simulink model "Commande_voiture_versionFinale2019"  (R2019b)
settings: Solver=ode1  StartTime=0.0  StopTime=inf  FixedStep=0.002  RelTol=1e-3  EnableMultiTasking=on
libraries: simulink x2, arduinolib x1
settings Model: SimulationMode=external  ExtModeTrigDuration=2  Creator=Alex  LastModifiedBy=franc
settings SolverCC: AutoInsertRateTranBlk=on
settings DataIOCC: SaveFormat=StructureWithTime  ReturnWorkspaceOutputs=off
settings OptimizationCC: PassReuseOutputArgsAs=Individual arguments  MaxStackSize=64  EfficientTunableParamExpr=on
settings DebuggingCC: ParameterPrecisionLossMsg=none  ParameterTunabilityLossMsg=error  ArithmeticOperatorsInVariantConditions=warning
settings HardwareCC: ProdBitPerInt=16  ProdBitPerPointer=16  ProdBitPerSizeT=16  ProdBitPerPtrDiffT=16  ProdLargestAtomicFloat=None  ProdWordSize=8  ProdHWDeviceType=Atmel->AVR
settings SFSimCC: SimUseLocalCustomCode=off  MATLABDynamicMemAlloc=off  CustomCodeUndefinedFunction=UseInterfaceOnly
settings RTWCC: SystemTargetFile=ert.tlc  HardwareBoard=Arduino Mega 2560  TLCOptions=-aInlineSetEventsForThisBaseRateFcn=TLC_FALSE -aSuppressMultiTaskScheduler=TLC_FALSE -aRateBasedStepFcn=1  TemplateMakefile=ert_default_tmf  RTWUseLocalCustomCode=off  Toolchain=Arduino AVR  BuildConfiguration=Faster Runs  IncludeHyperlinkInReport=on
settings CodeAppCC: ForceParamTrailComments=on  IgnoreCustomStorageClasses=off  OperatorAnnotations=on  SimulinkDataObjDesc=on  SFDataObjDesc=on  InsertBlockDesc=on
settings ERTTargetCC: SupportContinuousTime=on  SupportVariableSizeSignals=on

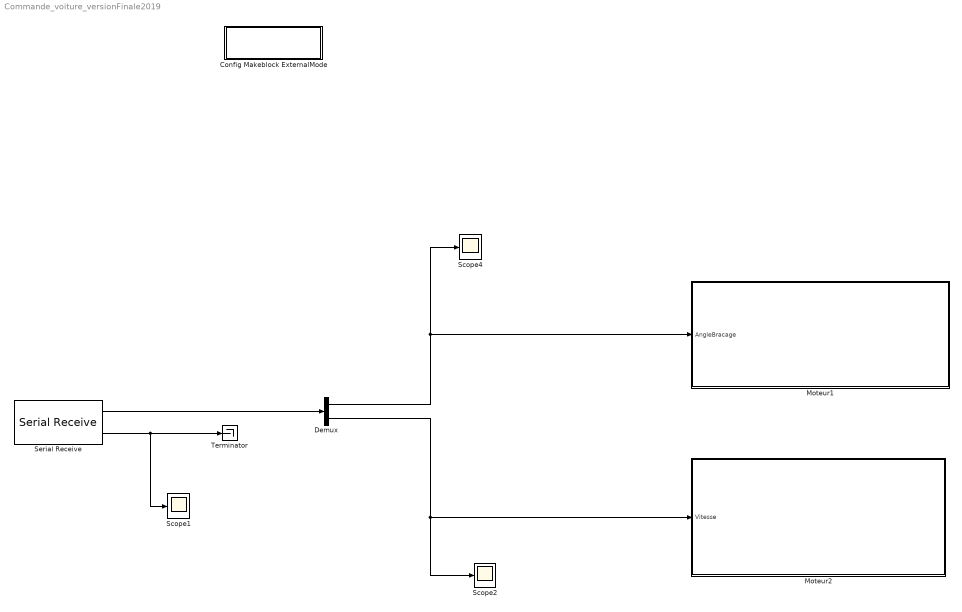
== system Commande_voiture_versionFinale2019 ==
  Config Makeblock ExternalMode : Subsystem  LoadFcn=set_param(gcb,'MaskHideContents','on')  InitFcn=|  TreatAsAtomicUnit=on
      | codertarget.arduinobase.registry.setBaudRate(gcs,115200)
      | set_param(gcb,'MaskHideContents','on')
      mask Display: disp('Makeblock external mode')
  Demux : Demux  Outputs=2
  Moteur1 : Subsystem
  Moteur2 : Subsystem
  Scope1 : Scope
  Scope2 : Scope
  Scope4 : Scope
  Serial Receive : arduinolib/Serial Receive  isARMArch=off  portNumber=2  DataType=int8  Datalength=2  SampleTime=0.1  showOutStatus=on  blockPlatform=arduino
      settings: SourceProductBaseCode=ARDUINO
  Terminator : Terminator
  wires:
  Serial Receive/2 -> Terminator/1, Scope1/1
  Serial Receive/1 -> Demux/1
  Demux/2 -> Scope2/1, Moteur2/1(Vitesse)
  Demux/1 -> Scope4/1, Moteur1/1(AngleBracage)

== system Commande_voiture_versionFinale2019/Config Makeblock ExternalMode ==

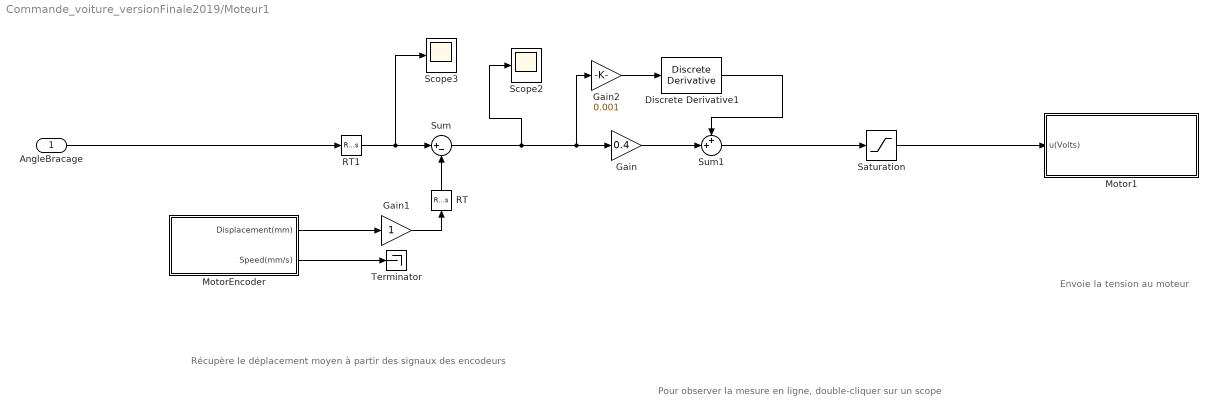
== system Commande_voiture_versionFinale2019/Moteur1 ==
  note: Pour observer la mesure en ligne, double-cliquer sur un scope
  note: Envoie la tension au moteur
  note: Récupère le déplacement moyen à partir des signaux des encodeurs
  AngleBracage : Inport
  Discrete Derivative1 : simulink/Discrete/Discrete Derivative  gainval=1.0  ICPrevScaledInput=0.0  OutMin=[]  OutMax=[]  OutDataType=fixdt(1, 16)  OutScaling=2^-10  DoSatur=off
  Gain : Gain  Gain=0.4
  Gain1 : Gain
  Gain2 : Gain  Gain=0.001
  Motor1 : Subsystem  mask{Vmax=12}
      mask prompts: Vmax "Power supply Voltage"
  MotorEncoder : Subsystem  mask{pulsePerTurn=8, beltPitch=1, nTeeth=40, gearRatio=75}
      mask prompts: pulsePerTurn "Encoder resolution"; beltPitch "Belt Pitch"; nTeeth "Number of teeth"; gearRatio "Gear ratio"
  RT : RateTransition  OutPortSampleTime=0.002
  RT1 : RateTransition  OutPortSampleTime=0.002
  Saturation : Saturate  UpperLimit=9  LowerLimit=-9
      settings: AttributesFormatString=[%<LowerLimit> %<UpperLimit>]
  Scope2 : Scope
  Scope3 : Scope
  Sum : Sum  Inputs=|+-
  Sum1 : Sum  Inputs=++|
  Terminator : Terminator
  wires:
  Gain1/1 -> RT/1
  Saturation/1 -> Motor1/1(u(Volts))
  RT/1 -> Sum/2
  MotorEncoder/1(Displacement(mm)) -> Gain1/1
  AngleBracage/1 -> RT1/1
  RT1/1 -> Scope3/1, Sum/1
  Discrete Derivative1/1 -> Sum1/1
  Gain2/1 -> Discrete Derivative1/1
  Sum/1 -> Gain2/1, Gain/1, Scope2/1
  Gain/1 -> Sum1/2
  Sum1/1 -> Saturation/1
  MotorEncoder/2(Speed(mm/s)) -> Terminator/1

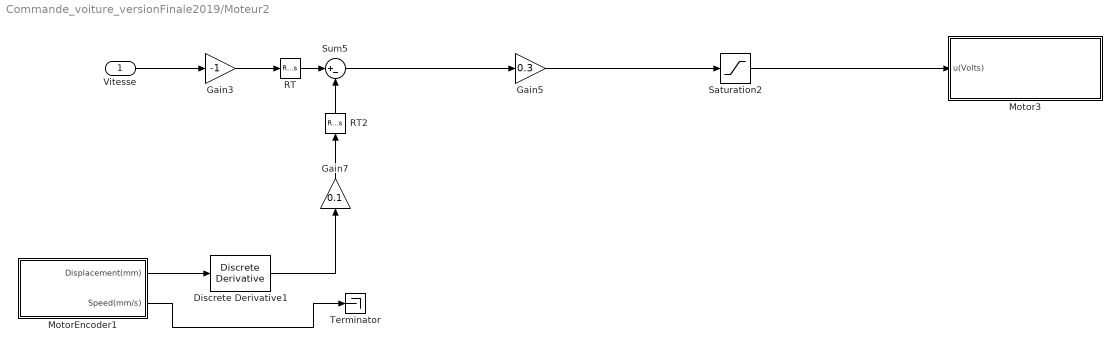
== system Commande_voiture_versionFinale2019/Moteur2 ==
  Vitesse : Inport
  Discrete Derivative1 : simulink/Discrete/Discrete Derivative  gainval=1.0  ICPrevScaledInput=0.0  OutMin=[]  OutMax=[]  OutDataType=fixdt(1, 16)  OutScaling=2^-10  DoSatur=off
  Gain3 : Gain  Gain=-1
  Gain5 : Gain  Gain=0.3
  Gain7 : Gain  Gain=0.1
  Motor3 : Subsystem  mask{Vmax=12}
      mask prompts: Vmax "Power supply Voltage"
  MotorEncoder1 : Subsystem  mask{pulsePerTurn=8, beltPitch=1, nTeeth=40, gearRatio=46}
      mask prompts: pulsePerTurn "Encoder resolution"; beltPitch "Belt Pitch"; nTeeth "Number of teeth"; gearRatio "Gear ratio"
  RT : RateTransition  OutPortSampleTime=0.002
  RT2 : RateTransition  OutPortSampleTime=0.002
  Saturation2 : Saturate  UpperLimit=9  LowerLimit=-9
      settings: AttributesFormatString=[%<LowerLimit> %<UpperLimit>]
  Sum5 : Sum  Inputs=|+-
  Terminator : Terminator
  wires:
  Saturation2/1 -> Motor3/1(u(Volts))
  Discrete Derivative1/1 -> Gain7/1
  Sum5/1 -> Gain5/1
  Gain5/1 -> Saturation2/1
  Gain3/1 -> RT/1
  MotorEncoder1/1(Displacement(mm)) -> Discrete Derivative1/1
  RT2/1 -> Sum5/2
  Gain7/1 -> RT2/1
  Vitesse/1 -> Gain3/1
  MotorEncoder1/2(Speed(mm/s)) -> Terminator/1
  RT/1 -> Sum5/1

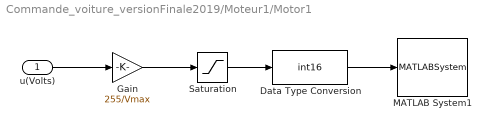
== system Commande_voiture_versionFinale2019/Moteur1/Motor1 ==
  u(Volts) : Inport
  Data Type Conversion : DataTypeConversion  OutDataTypeStr=int16
  Gain : Gain  Gain=255/Vmax
      settings: AttributesFormatString=%<Gain>
  MATLAB System1 : MATLABSystem  System=DCMotor1Set
      mask Type: DCMotor1Set
      mask Display:
      | disp('DC Motor 1');
      | port_label('input',1,'u');
  Saturation : Saturate  UpperLimit=255  LowerLimit=-255
  wires:
  Gain/1 -> Saturation/1
  u(Volts)/1 -> Gain/1
  Data Type Conversion/1 -> MATLAB System1/1
  Saturation/1 -> Data Type Conversion/1

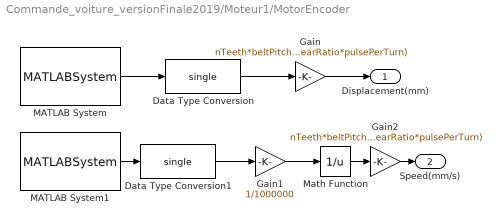
== system Commande_voiture_versionFinale2019/Moteur1/MotorEncoder ==
  Data Type Conversion : DataTypeConversion  OutDataTypeStr=single
  Data Type Conversion1 : DataTypeConversion  OutDataTypeStr=single
  Gain : Gain  Gain=nTeeth*beltPitch/(gearRatio*pulsePerTurn)  OutDataTypeStr=single
      settings: AttributesFormatString=%<Gain>
  Gain1 : Gain  Gain=1/1000000
  Gain2 : Gain  Gain=nTeeth*beltPitch/(gearRatio*pulsePerTurn)  OutDataTypeStr=single
      settings: AttributesFormatString=%<Gain>
  MATLAB System : MATLABSystem  System=Enc1Read  SampleTime=0.002
      mask Type: Enc1Read
      mask Display:
      | disp('Encoder 1');
      | port_label('output',1,'y');
  MATLAB System1 : MATLABSystem  System=Enc1Period  SampleTime=0.002
      mask Type: Enc1Period
      mask Display:
      | disp('Encoder Period 1');
      | port_label('output',1,'y');
  Math Function : Math  Operator=reciprocal  SignedPower=on  OutputSignalType=real  OutDataTypeStr=single
  Displacement(mm) : Outport  VectorParamsAs1DForOutWhenUnconnected=off
  Speed(mm/s) : Outport  Port=2  VectorParamsAs1DForOutWhenUnconnected=off
  wires:
  MATLAB System/1 -> Data Type Conversion/1
  Gain/1 -> Displacement(mm)/1
  Data Type Conversion/1 -> Gain/1
  Gain1/1 -> Math Function/1
  Data Type Conversion1/1 -> Gain1/1
  MATLAB System1/1 -> Data Type Conversion1/1
  Math Function/1 -> Gain2/1
  Gain2/1 -> Speed(mm/s)/1

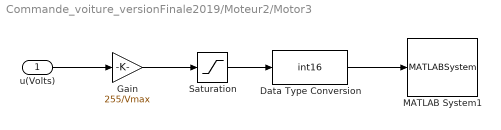
== system Commande_voiture_versionFinale2019/Moteur2/Motor3 ==
  u(Volts) : Inport
  Data Type Conversion : DataTypeConversion  OutDataTypeStr=int16
  Gain : Gain  Gain=255/Vmax
      settings: AttributesFormatString=%<Gain>
  MATLAB System1 : MATLABSystem  System=DCMotor2Set
      mask Type: DCMotor2Set
      mask Display:
      | disp('DC Motor 2');
      | port_label('input',1,'u');
  Saturation : Saturate  UpperLimit=255  LowerLimit=-255
  wires:
  Gain/1 -> Saturation/1
  u(Volts)/1 -> Gain/1
  Data Type Conversion/1 -> MATLAB System1/1
  Saturation/1 -> Data Type Conversion/1

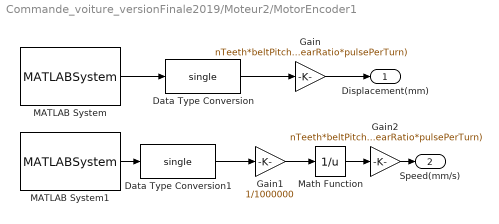
== system Commande_voiture_versionFinale2019/Moteur2/MotorEncoder1 ==
  Data Type Conversion : DataTypeConversion  OutDataTypeStr=single
  Data Type Conversion1 : DataTypeConversion  OutDataTypeStr=single
  Gain : Gain  Gain=nTeeth*beltPitch/(gearRatio*pulsePerTurn)  OutDataTypeStr=single
      settings: AttributesFormatString=%<Gain>
  Gain1 : Gain  Gain=1/1000000
  Gain2 : Gain  Gain=nTeeth*beltPitch/(gearRatio*pulsePerTurn)  OutDataTypeStr=single
      settings: AttributesFormatString=%<Gain>
  MATLAB System : MATLABSystem  System=Enc2Read  SampleTime=0.002
      mask Type: Enc2Read
      mask Display:
      | disp('Encoder 2');
      | port_label('output',1,'y');
  MATLAB System1 : MATLABSystem  System=Enc1Period  SampleTime=0.002
      mask Type: Enc1Period
      mask Display:
      | disp('Encoder Period 1');
      | port_label('output',1,'y');
  Math Function : Math  Operator=reciprocal  SignedPower=on  OutputSignalType=real  OutDataTypeStr=single
  Displacement(mm) : Outport  VectorParamsAs1DForOutWhenUnconnected=off
  Speed(mm/s) : Outport  Port=2  VectorParamsAs1DForOutWhenUnconnected=off
  wires:
  MATLAB System/1 -> Data Type Conversion/1
  Gain/1 -> Displacement(mm)/1
  Data Type Conversion/1 -> Gain/1
  Gain1/1 -> Math Function/1
  Data Type Conversion1/1 -> Gain1/1
  MATLAB System1/1 -> Data Type Conversion1/1
  Math Function/1 -> Gain2/1
  Gain2/1 -> Speed(mm/s)/1
